simulink model "plat_model"  (R2019a)
settings: Solver=FixedStepAuto  StartTime=0.0  StopTime=20  RelTol=1e-3  EnableMultiTasking=on
undefined symbols (not defined in the file or in its folder): Pull, up
libraries: speedgoatlib_IO183 x4, slrtlib x2
settings Model: Creator=vnalam  LastModifiedBy=vnalam
settings SolverCC: ConcurrentTasks=on  AutoInsertRateTranBlk=on
settings DataIOCC: SaveFormat=StructureWithTime
settings OptimizationCC: BlockReduction=off  OptimizeBlockIOStorage=off  BufferReuse=off  GlobalBufferReuse=off  ExpressionFolding=off  LocalBlockOutputs=off  OptimizeDataStoreBuffers=off  BusAssignmentInplaceUpdate=off
settings HardwareCC: ProdBitPerPointer=32  ProdBitPerSizeT=32  ProdBitPerPtrDiffT=32  ProdLargestAtomicFloat=None  ProdWordSize=32  ProdLongLongMode=on  ProdHWDeviceType=Generic->32-bit x86 compatible
settings RTWCC: SystemTargetFile=slrt.tlc  TemplateMakefile=slrt_default_tmf  Description=Simulink Real-Time  CodeExecutionProfiling=on  RTWCompilerOptimization=on
settings SimulinkRealTimeCC: SupportVariableSizeSignals=on  PreserveStateflowLocalDataDimensions=off  RL32LogTETModifier=off  xPCisDownloadable=off  xPCConcurrentTasks=on

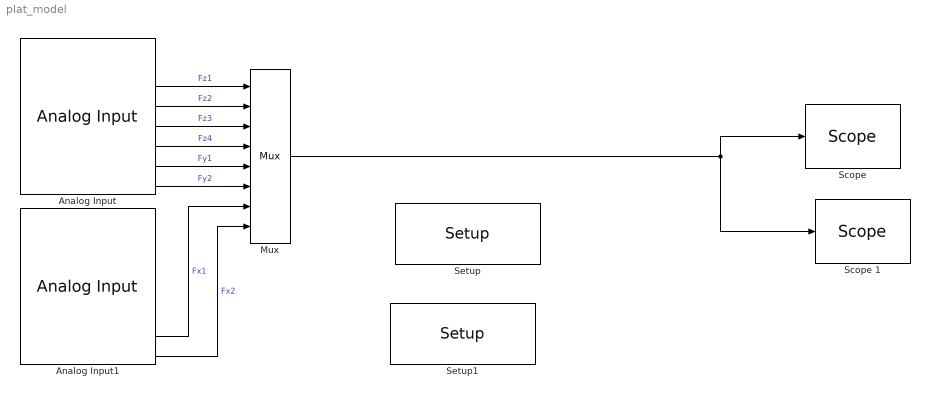
== system plat_model ==
  Analog Input : speedgoatlib_IO183/Analog Input  Priority=0  parModuleId=1  parSampTime=Ts  parPciSlot=-1  parAdChannelLow=1  parAdChannelHigh=8
      settings: SourceProductName=Simulink Real-Time: Speedgoat Library
  Analog Input1 : speedgoatlib_IO183/Analog Input  Priority=0  parModuleId=2  parSampTime=-1  parPciSlot=-1  parAdChannelLow=1  parAdChannelHigh=8
      settings: SourceProductName=Simulink Real-Time: Speedgoat Library
  Mux : Mux  Inputs=8
      settings: DisplayOption=signals
  "Scope " : slrtlib/Displays and Logging/Scope   scopeno=1  scopetype=Target  autostart=on  viewmode=Graphical rolling  formatstr='%15.6f'  grid=on  ylimits=[0,0]  nosamples=40000  noprepostsamples=0  interleave=1  triggermode=FreeRun  triggersignal=1  trigsignalfromport=off  triggerlevel=0.0  triggerslope=Either  triggerscope=1  triggersample=0  filename=data.dat  mode=Lazy  writesize=512  autorestart=off  dynamicfilemode=off  maxwritefilesize=512*1024^2
  Scope 1 : slrtlib/Displays and Logging/Scope   scopeno=2  scopetype=File  autostart=on  viewmode=Graphical redraw  formatstr='%15.6f'  grid=on  ylimits=[0,0]  nosamples=80000  noprepostsamples=0  interleave=1  triggermode=FreeRun  triggersignal=1  trigsignalfromport=off  triggerlevel=0.0  triggerslope=Either  triggerscope=1  triggersample=0  filename=pbase.dat  mode=Commit  writesize=512  autorestart=off  dynamicfilemode=off  maxwritefilesize=512*1024^2
  Setup : speedgoatlib_IO183/Setup  parModuleId=1  parPciSlot=-1  parDaSimult=on  parAdCoupling=Single Ended  parAdRange=+-10V  parAdChannelLow=1  parAdChannelHigh=8  parDaChannels=[1:4]  parDaRange=0..5V  parDaInit=[0]  parDaReset=[0]  parDoChannels=[1:8]  parDoInit=[0]  parDoReset=[1]  parDiChannels=[9:16]  parIOPullReferenceFront=Pull-up (3.3V)  parIOPullReferenceRear=Pull-up (3.3V)
      settings: SourceProductName=Simulink Real-Time: Speedgoat Library
  Setup1 : speedgoatlib_IO183/Setup  parModuleId=2  parPciSlot=-1  parDaSimult=on  parAdCoupling=Single Ended  parAdRange=+-10V  parAdChannelLow=1  parAdChannelHigh=8  parDaChannels=[1:4]  parDaRange=0..5V  parDaInit=[0]  parDaReset=[0]  parDoChannels=[1:8]  parDoInit=[0]  parDoReset=[1]  parDiChannels=[9:16]  parIOPullReferenceFront=Pull-up (3.3V)  parIOPullReferenceRear=Pull-up (3.3V)
      settings: SourceProductName=Simulink Real-Time: Speedgoat Library
  wires:
  Mux/1 -> "Scope "/1, Scope 1/1
  Analog Input/3 -> Mux/1  "Fz1"
  Analog Input/4 -> Mux/2  "Fz2"
  Analog Input/5 -> Mux/3  "Fz3"
  Analog Input/6 -> Mux/4  "Fz4"
  Analog Input/7 -> Mux/5  "Fy1"
  Analog Input/8 -> Mux/6  "Fy2"
  Analog Input1/7 -> Mux/7  "Fx1"
  Analog Input1/8 -> Mux/8  "Fx2"
